simulink model "subsistema_electromagnetico"  (R2024b)
settings: Solver=VariableStepAuto  StartTime=0.0  StopTime=10.0  RelTol=1e-3
values from neighbouring files (symbols this model uses):
  L_d = 6.6 * 10^-3    (= 0.0066)    [parametros.m]
  L_ls = 0.8 * 10^-3    (= 0.0008)    [parametros.m]
  L_q = 5.8 * 10^-3    (= 0.0058)    [parametros.m]
  lambda_m = 0.016    [parametros.m]
  P_p = 3    [parametros.m]
settings Model: Creator=nsorr  LastModifiedBy=nsorr

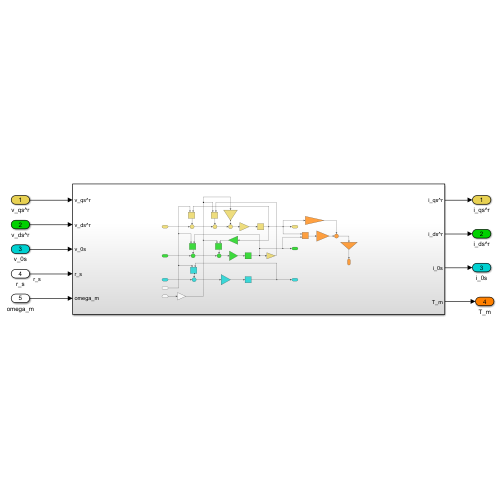
[thumbnail: Simulink's stored preview of the top-level diagram]
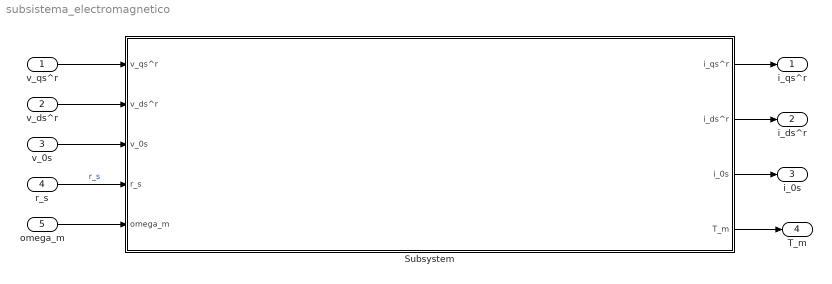
== system subsistema_electromagnetico ==
  v_qs^r : Inport
  v_ds^r : Inport  Port=2
  v_0s : Inport  Port=3
  r_s : Inport  Port=4
  omega_m : Inport  Port=5
  Subsystem : Subsystem
  i_qs^r : Outport
  i_ds^r : Outport  Port=2
  i_0s : Outport  Port=3
  T_m : Outport  Port=4
  wires:
  v_qs^r/1 -> Subsystem/1(v_qs^r)
  v_ds^r/1 -> Subsystem/2(v_ds^r)
  v_0s/1 -> Subsystem/3(v_0s)
  r_s/1 -> Subsystem/4(r_s)  "r_s"
  omega_m/1 -> Subsystem/5(omega_m)
  Subsystem/1(i_qs^r) -> i_qs^r/1
  Subsystem/2(i_ds^r) -> i_ds^r/1
  Subsystem/3(i_0s) -> i_0s/1
  Subsystem/4(T_m) -> T_m/1

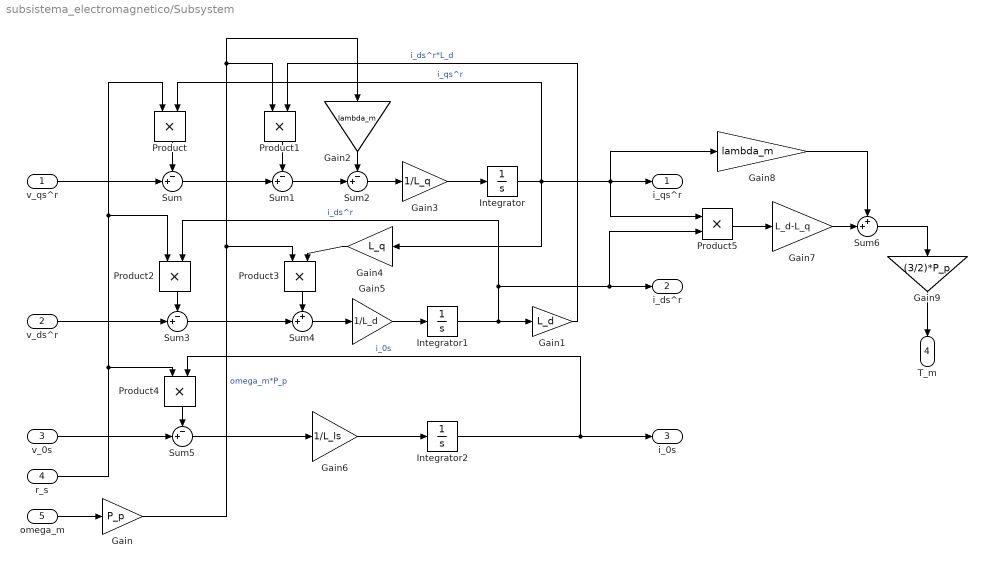
== system subsistema_electromagnetico/Subsystem ==
  v_qs^r : Inport
  v_ds^r : Inport  Port=2
  v_0s : Inport  Port=3
  r_s : Inport  Port=4
  omega_m : Inport  Port=5
  Gain : Gain  Gain=P_p
  Gain1 : Gain  Gain=L_d
  Gain2 : Gain  Gain=lambda_m
  Gain3 : Gain  Gain=1/L_q
  Gain4 : Gain  Gain=L_q
  Gain5 : Gain  Gain=1/L_d
  Gain6 : Gain  Gain=1/L_ls
  Gain7 : Gain  Gain=L_d-L_q
  Gain8 : Gain  Gain=lambda_m
  Gain9 : Gain  Gain=(3/2)*P_p
  Integrator : Integrator
  Integrator1 : Integrator
  Integrator2 : Integrator
  Product{,1..5} (6 alike) : Product
  Sum{,1..3,5} (5 alike) : Sum  Inputs=-+|
  Sum4 : Sum  Inputs=++|
  Sum6 : Sum  Inputs=++|
  i_qs^r : Outport
  i_ds^r : Outport  Port=2
  i_0s : Outport  Port=3
  T_m : Outport  Port=4
  wires:
  v_ds^r/1 -> Sum3/2
  Gain2/1 -> Sum2/1
  Sum6/1 -> Gain9/1
  Product/1 -> Sum/1
  v_qs^r/1 -> Sum/2
  Sum/1 -> Sum1/2
  Gain7/1 -> Sum6/2
  omega_m/1 -> Gain/1
  Gain/1 -> Gain2/1, Product1/1, Product3/1  "omega_m*P_p"
  Integrator2/1 -> i_0s/1, Product4/2  "i_0s"
  Product5/1 -> Gain7/1
  Integrator1/1 -> Product2/2, i_ds^r/1, Product5/2, Gain1/1  "i_ds^r"
  Gain8/1 -> Sum6/1
  Product3/1 -> Sum4/1
  v_0s/1 -> Sum5/2
  Gain9/1 -> T_m/1
  Gain3/1 -> Integrator/1
  Sum2/1 -> Gain3/1
  Integrator/1 -> i_qs^r/1, Gain8/1, Product5/1, Product/2, Gain4/1  "i_qs^r"
  r_s/1 -> Product4/1, Product/1, Product2/1
  Sum4/1 -> Gain5/1
  Sum1/1 -> Sum2/2
  Gain5/1 -> Integrator1/1
  Gain4/1 -> Product3/2
  Sum3/1 -> Sum4/2
  Product4/1 -> Sum5/1
  Product2/1 -> Sum3/1
  Gain1/1 -> Product1/2  "i_ds^r*L_d"
  Gain6/1 -> Integrator2/1
  Sum5/1 -> Gain6/1
  Product1/1 -> Sum1/1
